simulink model "PC_MSFS_STATION"  (R2021b)
settings: Solver=FixedStepAuto  StartTime=0.0  StopTime=700  FixedStep=0.03  RelTol=1e-3
undefined symbols (not defined in the file): DiscIntNeverNeededParam, f, MODEL, MODEL_INI
libraries: SimConnectToolbox x13, simulink x5, instrumentlib x3
(part 1 of 2)
settings Model: Creator=Andreas  LastModifiedBy=ae-dagbeyibor3
settings SolverCC: AlgebraicLoopSolver=TrustRegion
settings DebuggingCC: InheritedTsInSrcMsg=none  SFMachineParentedDataDiag=warning

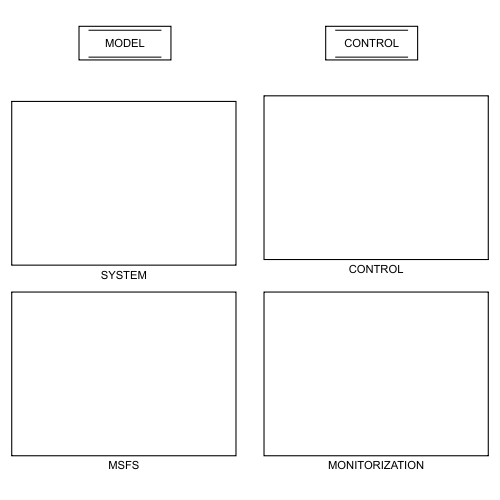
[thumbnail: Simulink's stored preview of the top-level diagram]
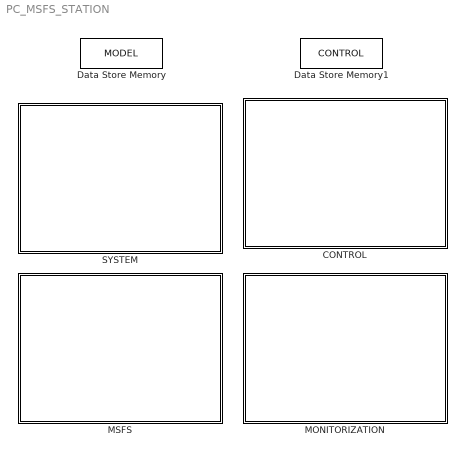
== system PC_MSFS_STATION ==
  CONTROL : Subsystem
  Data Store Memory : DataStoreMemory  DataStoreName=MODEL  ReadBeforeWriteMsg=warning  WriteAfterWriteMsg=warning  WriteAfterReadMsg=warning  InitialValue=MODEL_INI  ShowAdditionalParam=off  OutDataTypeStr=Bus: MODEL_Bus
  Data Store Memory1 : DataStoreMemory  DataStoreName=CONTROL  ReadBeforeWriteMsg=warning  WriteAfterWriteMsg=warning  WriteAfterReadMsg=warning  InitialValue=CONTROL_INI  ShowAdditionalParam=off  OutDataTypeStr=Bus: CONTROL_Bus
  MONITORIZATION : Subsystem
  MSFS : Subsystem
  SYSTEM : Subsystem

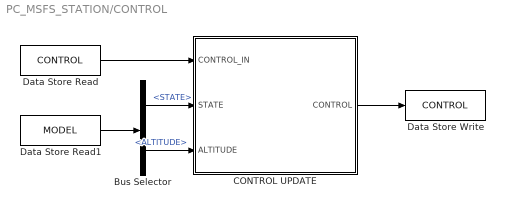
== system PC_MSFS_STATION/CONTROL ==
  Bus Selector : BusSelector  OutputSignals=STATE,INPUT.ALTITUDE
  CONTROL UPDATE : MATLAB Function  TreatAsAtomicUnit=on
  Data Store Read : DataStoreRead  DataStoreName=CONTROL  SampleTime=MODEL_INI.PARAM.SIM_SAMPLING_TIME  IndexOptions=Index vector (dialog)  Indices=1  OutputSizes=1
  Data Store Read1 : DataStoreRead  DataStoreName=MODEL  SampleTime=MODEL_INI.PARAM.SIM_SAMPLING_TIME  IndexOptions=Index vector (dialog)  Indices=1  OutputSizes=1
  Data Store Write : DataStoreWrite  DataStoreName=CONTROL  IndexOptions=Index vector (dialog)  Indices=1  OutputSizes=1
  wires:
  Data Store Read/1 -> CONTROL UPDATE/1(CONTROL_IN)
  CONTROL UPDATE/1(CONTROL) -> Data Store Write/1
  Bus Selector/1 -> CONTROL UPDATE/2(STATE)  "<STATE>"
  Data Store Read1/1 -> Bus Selector/1
  Bus Selector/2 -> CONTROL UPDATE/3(ALTITUDE)  "<ALTITUDE>"

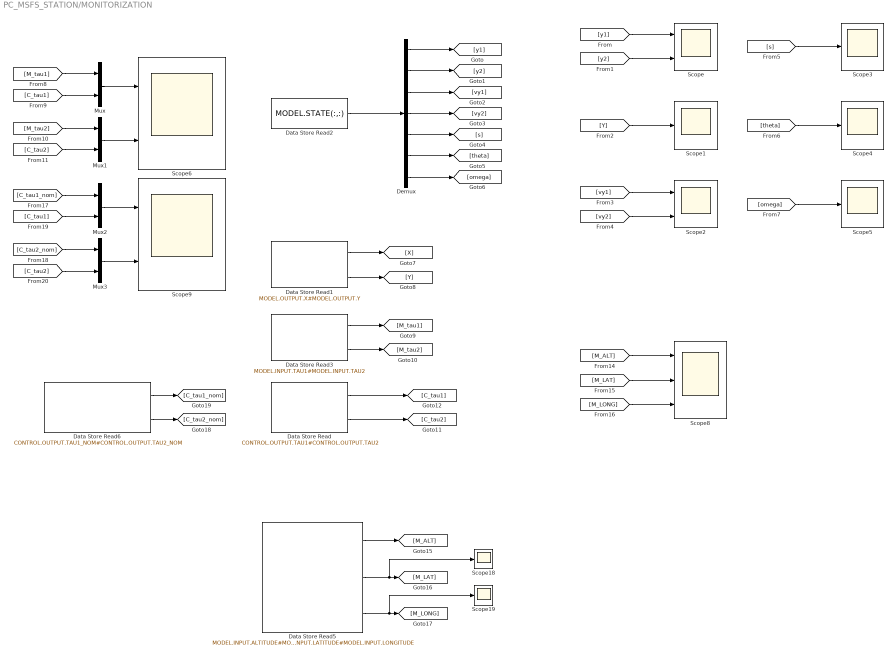
== system PC_MSFS_STATION/MONITORIZATION ==
  Data Store Read : DataStoreRead  DataStoreName=CONTROL  DataStoreElements=CONTROL.OUTPUT.TAU1#CONTROL.OUTPUT.TAU2  IndexOptions=Index vector (dialog)  Indices=1  OutputSizes=1
  Data Store Read1 : DataStoreRead  DataStoreName=MODEL  SampleTime=MODEL_INI.PARAM.SIM_SAMPLING_TIME  DataStoreElements=MODEL.OUTPUT.X#MODEL.OUTPUT.Y  IndexOptions=Index vector (dialog)  Indices=1  OutputSizes=1
  Data Store Read2 : DataStoreRead  DataStoreName=MODEL  SampleTime=MODEL_INI.PARAM.SIM_SAMPLING_TIME  DataStoreElements=MODEL.STATE(:,:)  IndexOptions=Index vector (dialog)  Indices=1  OutputSizes=1
  Data Store Read3 : DataStoreRead  DataStoreName=MODEL  SampleTime=MODEL_INI.PARAM.SIM_SAMPLING_TIME  DataStoreElements=MODEL.INPUT.TAU1#MODEL.INPUT.TAU2  IndexOptions=Index vector (dialog)  Indices=1  OutputSizes=1
  Data Store Read5 : DataStoreRead  DataStoreName=MODEL  SampleTime=MODEL_INI.PARAM.SIM_SAMPLING_TIME  DataStoreElements=MODEL.INPUT.ALTITUDE#MODEL.INPUT.LATITUDE#MODEL.INPUT.LONGITUDE  IndexOptions=Index vector (dialog)  Indices=1  OutputSizes=1
  Data Store Read6 : DataStoreRead  DataStoreName=CONTROL  DataStoreElements=CONTROL.OUTPUT.TAU1_NOM#CONTROL.OUTPUT.TAU2_NOM  IndexOptions=Index vector (dialog)  Indices=1  OutputSizes=1
  Demux : Demux  Outputs=7
  Mux{,1..3} (4 alike) : Mux  Inputs=2
  Scope{,2,6,9} (4 alike) : Scope  NumInputPorts=2
  Scope{1,3..5,18..19} (6 alike) : Scope
  Scope8 : Scope  NumInputPorts=3
  wires:
  Data Store Read2/1 -> Demux/1
  Demux/1 -> [y1]
  Demux/2 -> [y2]
  Demux/3 -> [vy1]
  Demux/4 -> [vy2]
  Demux/5 -> [s]
  Demux/6 -> [theta]
  Demux/7 -> [omega]
  [y1] -> Scope/1
  [y2] -> Scope/2
  Data Store Read1/1 -> [X]
  Data Store Read1/2 -> [Y]
  [Y] -> Scope1/1
  [vy2] -> Scope2/2
  [vy1] -> Scope2/1
  [s] -> Scope3/1
  [theta] -> Scope4/1
  [omega] -> Scope5/1
  Data Store Read3/1 -> [M_tau1]
  Data Store Read3/2 -> [M_tau2]
  Data Store Read/1 -> [C_tau1]
  Data Store Read/2 -> [C_tau2]
  Mux/1 -> Scope6/1
  Mux1/1 -> Scope6/2
  [M_tau1] -> Mux/1
  [M_tau2] -> Mux1/1
  [C_tau2] -> Mux1/2
  [C_tau1] -> Mux/2
  Data Store Read5/2 -> Scope18/1, [M_LAT]
  Data Store Read5/1 -> [M_ALT]
  Data Store Read5/3 -> Scope19/1, [M_LONG]
  [M_LAT] -> Scope8/2
  [M_ALT] -> Scope8/1
  [M_LONG] -> Scope8/3
  Data Store Read6/2 -> [C_tau2_nom]
  Data Store Read6/1 -> [C_tau1_nom]
  [C_tau1] -> Mux2/2
  [C_tau2] -> Mux3/2
  [C_tau2_nom] -> Mux3/1
  [C_tau1_nom] -> Mux2/1
  Mux3/1 -> Scope9/2
  Mux2/1 -> Scope9/1

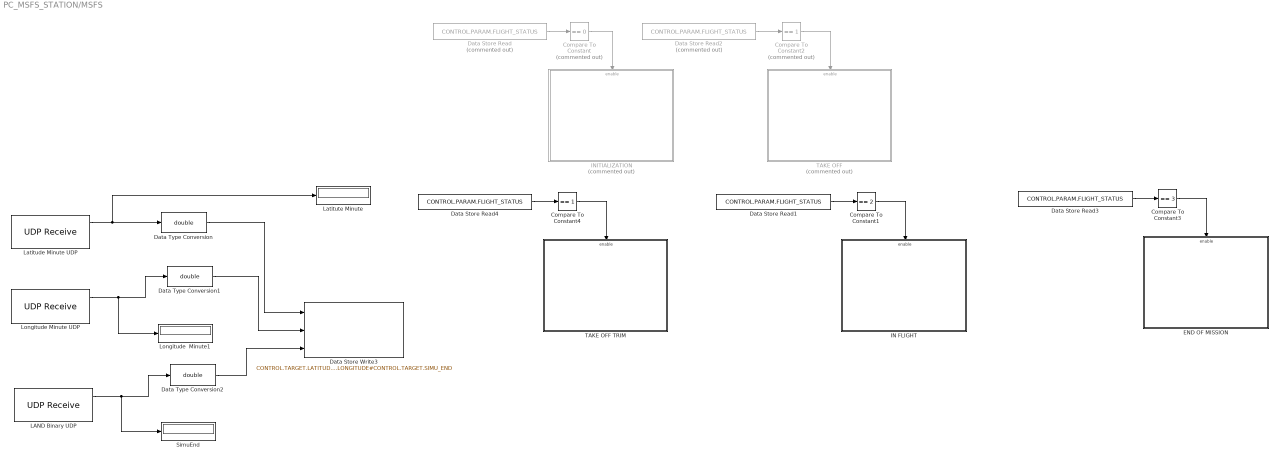
== system PC_MSFS_STATION/MSFS ==
  Compare To Constant : simulink/Logic and Bit Operations/Compare To Constant  Commented=on  relop===  const=0  OutDataTypeStr=boolean
  Compare To Constant1 : simulink/Logic and Bit Operations/Compare To Constant  relop===  const=2  OutDataTypeStr=boolean
  Compare To Constant2 : simulink/Logic and Bit Operations/Compare To Constant  Commented=on  relop===  const=1  OutDataTypeStr=boolean
  Compare To Constant3 : simulink/Logic and Bit Operations/Compare To Constant  relop===  const=3  OutDataTypeStr=boolean
  Compare To Constant4 : simulink/Logic and Bit Operations/Compare To Constant  relop===  const=1  OutDataTypeStr=boolean
  Data Store Read : DataStoreRead  Commented=on  DataStoreName=CONTROL  DataStoreElements=CONTROL.PARAM.FLIGHT_STATUS  IndexOptions=Index vector (dialog)  Indices=1  OutputSizes=1
  Data Store Read1 : DataStoreRead  DataStoreName=CONTROL  DataStoreElements=CONTROL.PARAM.FLIGHT_STATUS  IndexOptions=Index vector (dialog)  Indices=1  OutputSizes=1
  Data Store Read2 : DataStoreRead  Commented=on  DataStoreName=CONTROL  DataStoreElements=CONTROL.PARAM.FLIGHT_STATUS  IndexOptions=Index vector (dialog)  Indices=1  OutputSizes=1
  Data Store Read3 : DataStoreRead  DataStoreName=CONTROL  DataStoreElements=CONTROL.PARAM.FLIGHT_STATUS  IndexOptions=Index vector (dialog)  Indices=1  OutputSizes=1
  Data Store Read4 : DataStoreRead  DataStoreName=CONTROL  DataStoreElements=CONTROL.PARAM.FLIGHT_STATUS  IndexOptions=Index vector (dialog)  Indices=1  OutputSizes=1
  Data Store Write3 : DataStoreWrite  DataStoreName=CONTROL  DataStoreElements=CONTROL.TARGET.LATITUDE#CONTROL.TARGET.LONGITUDE#CONTROL.TARGET.SIMU_END  IndexOptions=Index vector (dialog)  Indices=1  OutputSizes=1
  Data Type Conversion : DataTypeConversion  OutDataTypeStr=double
  Data Type Conversion1 : DataTypeConversion  OutDataTypeStr=double
  Data Type Conversion2 : DataTypeConversion  OutDataTypeStr=double
  END OF MISSION : Subsystem
  IN FLIGHT : Subsystem
  INITIALIZATION : Subsystem  Commented=on
  LAND Binary UDP : instrumentlib/UDP Receive  Priority=1  Host=127.0.0.1  Port=8081  LocalPort=8086  EnablePortSharing=off  GetLatestData=off  DataSize=[1 1]  DataType=single  ASCIIFormatting=%f,  Terminator=LF  ByteOrder=BigEndian  EnableBlockingMode=off  Timeout=5  SampleTime=0.03  LocalAddress=127.0.0.1
  Latitude Minute UDP : instrumentlib/UDP Receive  Priority=1  Host=127.0.0.1  Port=8081  LocalPort=8082  EnablePortSharing=off  GetLatestData=off  DataSize=[1 1]  DataType=single  ASCIIFormatting=%f,  Terminator=LF  ByteOrder=BigEndian  EnableBlockingMode=off  Timeout=5  SampleTime=0.03  LocalAddress=127.0.0.1
  Latitute Minute : Display
  Longitude  Minute1 : Display
  Longitude Minute UDP : instrumentlib/UDP Receive  Priority=1  Host=127.0.0.1  Port=8081  LocalPort=8084  EnablePortSharing=off  GetLatestData=off  DataSize=[1 1]  DataType=single  ASCIIFormatting=%f,  Terminator=LF  ByteOrder=BigEndian  EnableBlockingMode=off  Timeout=5  SampleTime=0.03  LocalAddress=127.0.0.1
  SimuEnd : Display
  TAKE OFF : Subsystem  Commented=on
  TAKE OFF TRIM : Subsystem
  wires:
  Data Store Read/1 -> Compare To Constant/1
  Compare To Constant/1 -> INITIALIZATION/Enable
  Data Store Read1/1 -> Compare To Constant1/1
  Compare To Constant1/1 -> IN FLIGHT/Enable
  Data Store Read2/1 -> Compare To Constant2/1
  Compare To Constant2/1 -> TAKE OFF/Enable
  Compare To Constant3/1 -> END OF MISSION/Enable
  Data Store Read3/1 -> Compare To Constant3/1
  Data Store Read4/1 -> Compare To Constant4/1
  Compare To Constant4/1 -> TAKE OFF TRIM/Enable
  Longitude Minute UDP/1 -> Longitude  Minute1/1, Data Type Conversion1/1
  Data Type Conversion/1 -> Data Store Write3/1
  Latitude Minute UDP/1 -> Latitute Minute/1, Data Type Conversion/1
  Data Type Conversion1/1 -> Data Store Write3/2
  LAND Binary UDP/1 -> SimuEnd/1, Data Type Conversion2/1
  Data Type Conversion2/1 -> Data Store Write3/3

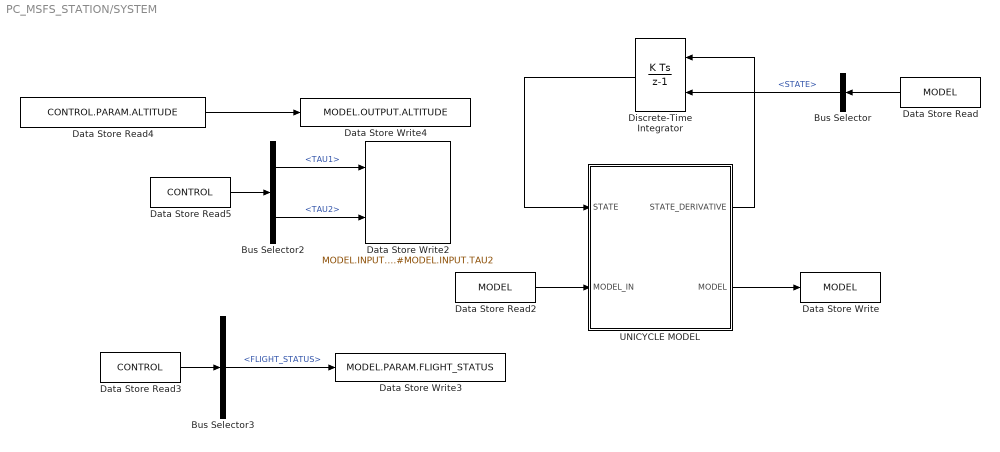
== system PC_MSFS_STATION/SYSTEM ==
  Bus Selector : BusSelector  OutputSignals=STATE
  Bus Selector2 : BusSelector  OutputSignals=OUTPUT.TAU1,OUTPUT.TAU2
  Bus Selector3 : BusSelector  OutputSignals=PARAM.FLIGHT_STATUS
  Data Store Read : DataStoreRead  DataStoreName=MODEL  SampleTime=MODEL_INI.PARAM.SIM_SAMPLING_TIME  IndexOptions=Index vector (dialog)  Indices=1  OutputSizes=1
  Data Store Read2 : DataStoreRead  DataStoreName=MODEL  SampleTime=MODEL_INI.PARAM.SIM_SAMPLING_TIME  IndexOptions=Index vector (dialog)  Indices=1  OutputSizes=1
  Data Store Read3 : DataStoreRead  DataStoreName=CONTROL  IndexOptions=Index vector (dialog)  Indices=1  OutputSizes=1
  Data Store Read4 : DataStoreRead  DataStoreName=CONTROL  DataStoreElements=CONTROL.PARAM.ALTITUDE  IndexOptions=Index vector (dialog)  Indices=1  OutputSizes=1
  Data Store Read5 : DataStoreRead  DataStoreName=CONTROL  IndexOptions=Index vector (dialog)  Indices=1  OutputSizes=1
  Data Store Write : DataStoreWrite  DataStoreName=MODEL  IndexOptions=Index vector (dialog)  Indices=1  OutputSizes=1
  Data Store Write2 : DataStoreWrite  DataStoreName=MODEL  DataStoreElements=MODEL.INPUT.TAU1#MODEL.INPUT.TAU2  IndexOptions=Index vector (dialog)  Indices=1  OutputSizes=1
  Data Store Write3 : DataStoreWrite  DataStoreName=MODEL  DataStoreElements=MODEL.PARAM.FLIGHT_STATUS  IndexOptions=Index vector (dialog)  Indices=1  OutputSizes=1
  Data Store Write4 : DataStoreWrite  DataStoreName=MODEL  DataStoreElements=MODEL.OUTPUT.ALTITUDE  IndexOptions=Index vector (dialog)  Indices=1  OutputSizes=1
  Discrete-Time Integrator : DiscreteIntegrator  InitialConditionSource=external  SampleTime=-1  ICPrevOutput=DiscIntNeverNeededParam  ICPrevScaledInput=DiscIntNeverNeededParam
  UNICYCLE MODEL : MATLAB Function  TreatAsAtomicUnit=on
  wires:
  Discrete-Time Integrator/1 -> UNICYCLE MODEL/1(STATE)
  UNICYCLE MODEL/1(STATE_DERIVATIVE) -> Discrete-Time Integrator/1
  Bus Selector/1 -> Discrete-Time Integrator/2  "<STATE>"
  Data Store Read/1 -> Bus Selector/1
  Data Store Read2/1 -> UNICYCLE MODEL/2(MODEL_IN)
  UNICYCLE MODEL/2(MODEL) -> Data Store Write/1
  Bus Selector2/2 -> Data Store Write2/2  "<TAU2>"
  Bus Selector2/1 -> Data Store Write2/1  "<TAU1>"
  Data Store Read5/1 -> Bus Selector2/1
  Data Store Read3/1 -> Bus Selector3/1
  Bus Selector3/1 -> Data Store Write3/1  "<FLIGHT_STATUS>"
  Data Store Read4/1 -> Data Store Write4/1

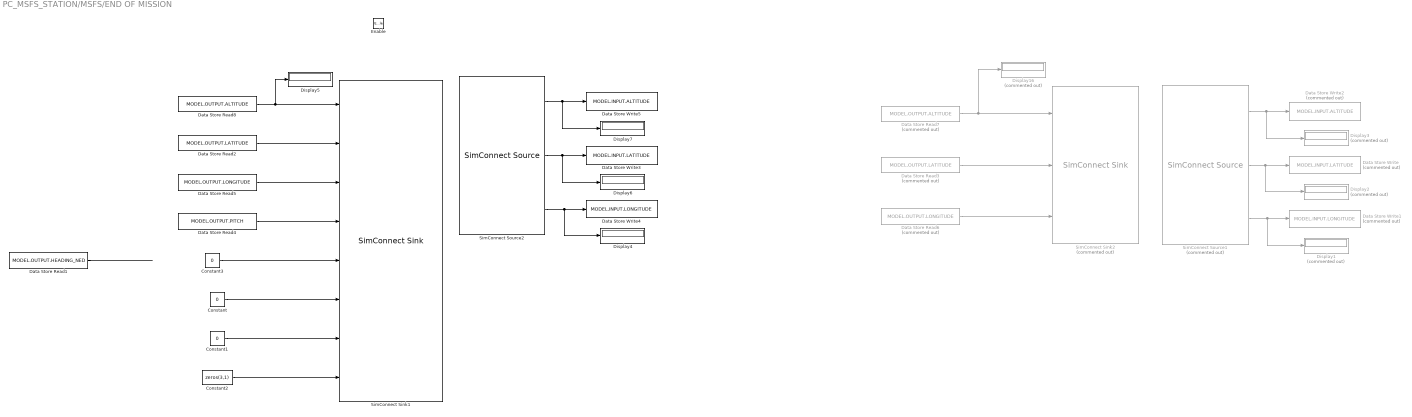
== system PC_MSFS_STATION/MSFS/END OF MISSION ==
  Enable : EnablePort
  Constant : Constant  Value=0  SampleTime=-1
  Constant1 : Constant  Value=0  SampleTime=-1
  Constant2 : Constant  Value=zeros(3,1)  SampleTime=-1
  Constant3 : Constant  Value=0  SampleTime=-1
  Data Store Read1 : DataStoreRead  DataStoreName=MODEL  DataStoreElements=MODEL.OUTPUT.HEADING_NED  IndexOptions=Index vector (dialog)  Indices=1  OutputSizes=1
  Data Store Read2 : DataStoreRead  DataStoreName=MODEL  DataStoreElements=MODEL.OUTPUT.LATITUDE  IndexOptions=Index vector (dialog)  Indices=1  OutputSizes=1
  Data Store Read3 : DataStoreRead  Commented=on  DataStoreName=MODEL  DataStoreElements=MODEL.OUTPUT.LATITUDE  IndexOptions=Index vector (dialog)  Indices=1  OutputSizes=1
  Data Store Read4 : DataStoreRead  DataStoreName=MODEL  DataStoreElements=MODEL.OUTPUT.PITCH  IndexOptions=Index vector (dialog)  Indices=1  OutputSizes=1
  Data Store Read5 : DataStoreRead  DataStoreName=MODEL  DataStoreElements=MODEL.OUTPUT.LONGITUDE  IndexOptions=Index vector (dialog)  Indices=1  OutputSizes=1
  Data Store Read6 : DataStoreRead  Commented=on  DataStoreName=MODEL  DataStoreElements=MODEL.OUTPUT.LONGITUDE  IndexOptions=Index vector (dialog)  Indices=1  OutputSizes=1
  Data Store Read7 : DataStoreRead  Commented=on  DataStoreName=MODEL  DataStoreElements=MODEL.OUTPUT.ALTITUDE  IndexOptions=Index vector (dialog)  Indices=1  OutputSizes=1
  Data Store Read8 : DataStoreRead  DataStoreName=MODEL  DataStoreElements=MODEL.OUTPUT.ALTITUDE  IndexOptions=Index vector (dialog)  Indices=1  OutputSizes=1
  Data Store Write : DataStoreWrite  Commented=on  DataStoreName=MODEL  DataStoreElements=MODEL.INPUT.LATITUDE  IndexOptions=Index vector (dialog)  Indices=1  OutputSizes=1
  Data Store Write1 : DataStoreWrite  Commented=on  DataStoreName=MODEL  DataStoreElements=MODEL.INPUT.LONGITUDE  IndexOptions=Index vector (dialog)  Indices=1  OutputSizes=1
  Data Store Write2 : DataStoreWrite  Commented=on  DataStoreName=MODEL  DataStoreElements=MODEL.INPUT.ALTITUDE  IndexOptions=Index vector (dialog)  Indices=1  OutputSizes=1
  Data Store Write3 : DataStoreWrite  DataStoreName=MODEL  DataStoreElements=MODEL.INPUT.LATITUDE  IndexOptions=Index vector (dialog)  Indices=1  OutputSizes=1
  Data Store Write4 : DataStoreWrite  DataStoreName=MODEL  DataStoreElements=MODEL.INPUT.LONGITUDE  IndexOptions=Index vector (dialog)  Indices=1  OutputSizes=1
  Data Store Write5 : DataStoreWrite  DataStoreName=MODEL  DataStoreElements=MODEL.INPUT.ALTITUDE  IndexOptions=Index vector (dialog)  Indices=1  OutputSizes=1
  Display{1..3,16} (4 alike) : Display  Commented=on
  Display{4..7} (4 alike) : Display
  SimConnect Sink1 : SimConnectToolbox/SimConnect Sink  configurationIndex=0  connectionName=SimConnectSink  variables=|
      | PLANE ALTITUDE, FEET;
      | PLANE LATITUDE, RADIANS;
      | PLANE LONGITUDE, RADIANS;
      | PLANE PITCH DEGREES, RADIANS;
      | PLANE HEADING DEGREES TRUE, RADIANS;
      | ROTATION VELOCITY BODY X, FEET PER SECOND;
      | AILERON POSITION, POSITION;
      | AILERON TRIM PCT, PERCENT;
      settings: SourceProductName=SimConnect Toolbox
      mask Display:
      | % This is a new mask on top of the base mask.
      | % Use "View base mask" link below to see the base mask.
      | %port_label('input', 1, 'Rudder Trim', 'texmode', 'on')
      | port_label('input', 1, 'PLANE ALTITUDE, FEET', 'texmode', 'on')
      | port_label('input', 2, 'PLANE LATITUDE, RADIANS', 'texmode', 'on')
      | port_label('input', 3, 'PLANE LONGITUDE, RADIANS', 'texmode', 'on')
      | port_label('input', 4, 'PITCH DEGREES, RADIANS', 'texmode', 'on')
      | port_label('input', 5, 'HEADING DEGREES TRUE, RADIANS', 'texmode', 'on')
      | port_label('input', 6, 'VELOCITY BODY X, FEET PER SECOND', 'texmode', 'on')
      | port_label('input', 7, 'AILERON POSITION, POSITION', 'texmode', 'on')
      | port_label('input', 8, 'AILERON TRIM PCT, PERCENT OVER 100', 'texmode', 'on')
  SimConnect Sink2 : SimConnectToolbox/SimConnect Sink  Commented=on  configurationIndex=0  connectionName=SimConnectSink  variables=|
      | PLANE ALTITUDE, FEET;
      | PLANE LATITUDE, RADIANS;
      | PLANE LONGITUDE, RADIANS;
      settings: SourceProductName=SimConnect Toolbox
      mask Display:
      | % This is a new mask on top of the base mask.
      | % Use "View base mask" link below to see the base mask.
      | %port_label('input', 1, 'Rudder Trim', 'texmode', 'on')
      | port_label('input', 1, 'PLANE ALTITUDE, FEET', 'texmode', 'on')
      | port_label('input', 2, 'PLANE LATITUDE, RADIANS', 'texmode', 'on')
      | port_label('input', 3, 'PLANE LONGITUDE, RADIANS', 'texmode', 'on')
  SimConnect Source1 : SimConnectToolbox/SimConnect Source  Commented=on  configurationIndex=0  connectionName=SimConnectSource  variables=|
      | PLANE ALTITUDE, FEET;
      | PLANE LATITUDE, RADIANS;
      | PLANE LONGITUDE, RADIANS;
      settings: SourceProductName=SimConnect Toolbox
      mask Display:
      | % This is a new mask on top of the base mask.
      | % Use "View base mask" link below to see the base mask.
      | % port_label('output', 1, 'g', 'texmode', 'on')
      | port_label('output', 1, 'PLANE ALTITUDE, FEET', 'texmode', 'on')
      | port_label('output', 2, 'PLANE LATITUDE, RADIANS', 'texmode', 'on')
      | port_label('output', 3, 'PLANE LONGITUDE, RADIANS', 'texmode', 'on')
  SimConnect Source2 : SimConnectToolbox/SimConnect Source  configurationIndex=0  connectionName=SimConnectSource  variables=|
      | PLANE ALTITUDE, FEET;
      | PLANE LATITUDE, RADIANS;
      | PLANE LONGITUDE, RADIANS;
      settings: SourceProductName=SimConnect Toolbox
      mask Display:
      | % This is a new mask on top of the base mask.
      | % Use "View base mask" link below to see the base mask.
      | % port_label('output', 1, 'g', 'texmode', 'on')
      | port_label('output', 1, 'PLANE ALTITUDE, FEET', 'texmode', 'on')
      | port_label('output', 2, 'PLANE LATITUDE, RADIANS', 'texmode', 'on')
      | port_label('output', 3, 'PLANE LONGITUDE, RADIANS', 'texmode', 'on')
  wires:
  SimConnect Source1/3 -> Data Store Write1/1, Display1/1
  SimConnect Source1/1 -> Data Store Write2/1, Display3/1
  SimConnect Source1/2 -> Display2/1, Data Store Write/1
  Data Store Read7/1 -> Display16/1, SimConnect Sink2/1
  Data Store Read6/1 -> SimConnect Sink2/3
  Data Store Read3/1 -> SimConnect Sink2/2
  SimConnect Source2/1 -> Display7/1, Data Store Write5/1
  Data Store Read5/1 -> SimConnect Sink1/3
  Data Store Read2/1 -> SimConnect Sink1/2
  Data Store Read8/1 -> SimConnect Sink1/1, Display5/1
  SimConnect Source2/2 -> Data Store Write3/1, Display6/1
  Data Store Read4/1 -> SimConnect Sink1/4
  SimConnect Source2/3 -> Display4/1, Data Store Write4/1
  Constant1/1 -> SimConnect Sink1/7
  Data Store Read1/1 -> ?
  Constant2/1 -> SimConnect Sink1/8
  Constant/1 -> SimConnect Sink1/6
  Constant3/1 -> SimConnect Sink1/5

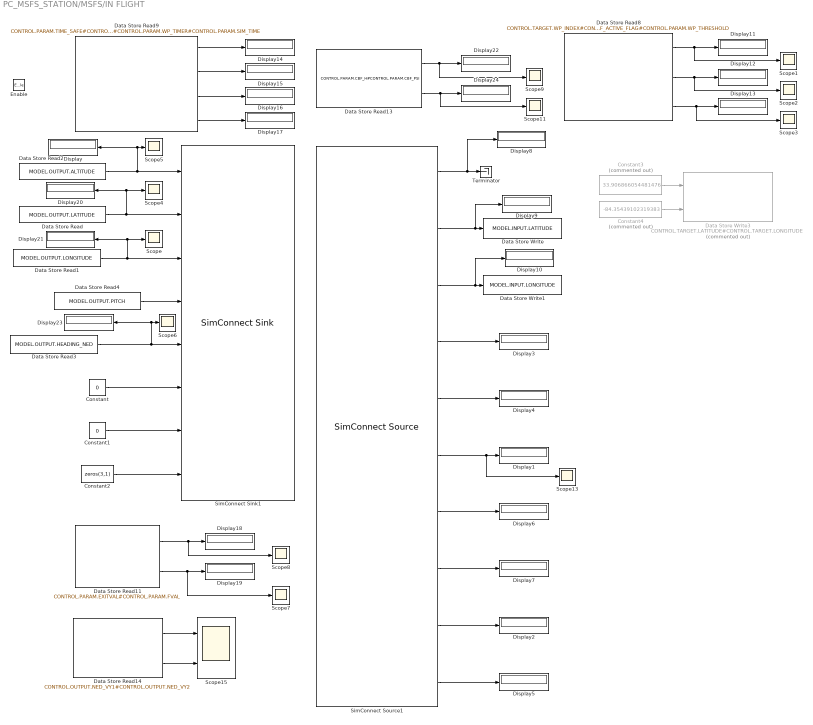
== system PC_MSFS_STATION/MSFS/IN FLIGHT ==
  Enable : EnablePort
  Constant : Constant  Value=0  SampleTime=-1
  Constant1 : Constant  Value=0  SampleTime=-1
  Constant2 : Constant  Value=zeros(3,1)  SampleTime=-1
  Constant3 : Constant  Commented=on  Value=33.906866054481476  SampleTime=-1
  Constant4 : Constant  Commented=on  Value=-84.35439102319383  SampleTime=-1
  Data Store Read : DataStoreRead  DataStoreName=MODEL  DataStoreElements=MODEL.OUTPUT.LATITUDE  IndexOptions=Index vector (dialog)  Indices=1  OutputSizes=1
  Data Store Read1 : DataStoreRead  DataStoreName=MODEL  DataStoreElements=MODEL.OUTPUT.LONGITUDE  IndexOptions=Index vector (dialog)  Indices=1  OutputSizes=1
  Data Store Read11 : DataStoreRead  DataStoreName=CONTROL  DataStoreElements=CONTROL.PARAM.EXITVAL#CONTROL.PARAM.FVAL  IndexOptions=Index vector (dialog)  Indices=1  OutputSizes=1
  Data Store Read13 : DataStoreRead  DataStoreName=CONTROL  DataStoreElements=CONTROL.PARAM.CBF_H#CONTROL.PARAM.CBF_PSI  IndexOptions=Index vector (dialog)  Indices=1  OutputSizes=1
  Data Store Read14 : DataStoreRead  DataStoreName=CONTROL  DataStoreElements=CONTROL.OUTPUT.NED_VY1#CONTROL.OUTPUT.NED_VY2  IndexOptions=Index vector (dialog)  Indices=1  OutputSizes=1
  Data Store Read2 : DataStoreRead  DataStoreName=MODEL  DataStoreElements=MODEL.OUTPUT.ALTITUDE  IndexOptions=Index vector (dialog)  Indices=1  OutputSizes=1
  Data Store Read3 : DataStoreRead  DataStoreName=MODEL  DataStoreElements=MODEL.OUTPUT.HEADING_NED  IndexOptions=Index vector (dialog)  Indices=1  OutputSizes=1
  Data Store Read4 : DataStoreRead  DataStoreName=MODEL  DataStoreElements=MODEL.OUTPUT.PITCH  IndexOptions=Index vector (dialog)  Indices=1  OutputSizes=1
  Data Store Read8 : DataStoreRead  DataStoreName=CONTROL  DataStoreElements=CONTROL.TARGET.WP_INDEX#CONTROL.PARAM.CBF_ACTIVE_FLAG#CONTROL.PARAM.WP_THRESHOLD  IndexOptions=Index vector (dialog)  Indices=1  OutputSizes=1
  Data Store Read9 : DataStoreRead  DataStoreName=CONTROL  DataStoreElements=CONTROL.PARAM.TIME_SAFE#CONTROL.PARAM.TIMER#CONTROL.PARAM.WP_TIMER#CONTROL.PARAM.SIM_TIME  IndexOptions=Index vector (dialog)  Indices=1  OutputSizes=1
  Data Store Write : DataStoreWrite  DataStoreName=MODEL  DataStoreElements=MODEL.INPUT.LATITUDE  IndexOptions=Index vector (dialog)  Indices=1  OutputSizes=1
  Data Store Write1 : DataStoreWrite  DataStoreName=MODEL  DataStoreElements=MODEL.INPUT.LONGITUDE  IndexOptions=Index vector (dialog)  Indices=1  OutputSizes=1
  Data Store Write3 : DataStoreWrite  Commented=on  DataStoreName=CONTROL  DataStoreElements=CONTROL.TARGET.LATITUDE#CONTROL.TARGET.LONGITUDE  IndexOptions=Index vector (dialog)  Indices=1  OutputSizes=1
  Display{,1..24} (25 alike) : Display
  Scope{,1..9,11,13} (12 alike) : Scope
  Scope15 : Scope  NumInputPorts=2
  SimConnect Sink1 : SimConnectToolbox/SimConnect Sink  configurationIndex=0  connectionName=SimConnectSink  variables=|
      | PLANE ALTITUDE, FEET;
      | PLANE LATITUDE, RADIANS;
      | PLANE LONGITUDE, RADIANS;
      | PLANE PITCH DEGREES, RADIANS;
      | PLANE HEADING DEGREES TRUE, RADIANS;
      | ROTATION VELOCITY BODY X, FEET PER SECOND;
      | AILERON POSITION, POSITION;
      | AILERON TRIM PCT, PERCENT;
      settings: SourceProductName=SimConnect Toolbox
      mask Display:
      | % This is a new mask on top of the base mask.
      | % Use "View base mask" link below to see the base mask.
      | %port_label('input', 1, 'Rudder Trim', 'texmode', 'on')
      | port_label('input', 1, 'PLANE ALTITUDE, FEET', 'texmode', 'on')
      | port_label('input', 2, 'PLANE LATITUDE, RADIANS', 'texmode', 'on')
      | port_label('input', 3, 'PLANE LONGITUDE, RADIANS', 'texmode', 'on')
      | port_label('input', 4, 'PITCH DEGREES, RADIANS', 'texmode', 'on')
      | port_label('input', 5, 'HEADING DEGREES TRUE, RADIANS', 'texmode', 'on')
      | port_label('input', 6, 'VELOCITY BODY X, FEET PER SECOND', 'texmode', 'on')
      | port_label('input', 7, 'AILERON POSITION, POSITION', 'texmode', 'on')
      | port_label('input', 8, 'AILERON TRIM PCT, PERCENT OVER 100', 'texmode', 'on')
  SimConnect Source1 : SimConnectToolbox/SimConnect Source  configurationIndex=0  connectionName=SimConnectSource  variables=|
      | PLANE ALTITUDE, FEET;
      | PLANE LATITUDE, RADIANS;
      | PLANE LONGITUDE, RADIANS;
      | ROTATION VELOCITY BODY X, FEET PER SECOND;
      | PLANE PITCH DEGREES, RADIANS;
      | PLANE HEADING DEGREES TRUE, RADIANS;
      | PLANE HEADING DEGREES MAGNETIC, RADIANS;
      | PLANE HEADING DEGREES GYRO, DEGREES;
      | AILERON POSITION, POSITION;
      | AILERON TRIM PCT, PERCENT OVER 100;
      settings: SourceProductName=SimConnect Toolbox
      mask Display:
      | % This is a new mask on top of the base mask.
      | % Use "View base mask" link below to see the base mask.
      | % port_label('output', 1, 'g', 'texmode', 'on')
      | port_label('output', 1, 'PLANE ALTITUDE, FEET', 'texmode', 'on')
      | port_label('output', 2, 'PLANE LATITUDE, RADIANS', 'texmode', 'on')
      | port_label('output', 3, 'PLANE LONGITUDE, RADIANS', 'texmode', 'on')
      | port_label('output', 4, 'VELOCITY BODY X, FEET PER SECOND', 'texmode', 'on')
      | port_label('output', 5, 'PITCH DEGREES, RADIANS', 'texmode', 'on')
      | port_label('output', 6, 'HEADING DEGREES TRUE, RADIANS', 'texmode', 'on')
      | port_label('output', 7, 'HEADING DEGREES MAGNETIC, RADIANS', 'texmode', 'on')
      | port_label('output', 8, 'HEADING DEGREES GYRO, DEGREES', 'texmode', 'on')
      | port_label('output', 9, 'AILERON POSITION, POSITION', 'texmode', 'on')
      | port_label('output', 10, 'AILERON TRIM PCT, PERCENT OVER 100', 'texmode', 'on')
  Terminator : Terminator
  wires:
  Constant2/1 -> SimConnect Sink1/8
  SimConnect Source1/9 -> Display2/1
  Constant/1 -> SimConnect Sink1/6
  Data Store Read1/1 -> Display21/1, Scope/1, SimConnect Sink1/3
  Constant1/1 -> SimConnect Sink1/7
  SimConnect Source1/5 -> Display4/1
  SimConnect Source1/3 -> Display10/1, Data Store Write1/1
  SimConnect Source1/2 -> Display9/1, Data Store Write/1
  SimConnect Source1/8 -> Display7/1
  SimConnect Source1/6 -> Scope13/1, Display1/1
  Data Store Read2/1 -> Display/1, Scope5/1, SimConnect Sink1/1
  Data Store Read/1 -> Display20/1, Scope4/1, SimConnect Sink1/2
  Data Store Read4/1 -> SimConnect Sink1/4
  SimConnect Source1/4 -> Display3/1
  SimConnect Source1/1 -> Terminator/1, Display8/1
  SimConnect Source1/7 -> Display6/1
  SimConnect Source1/10 -> Display5/1
  Data Store Read9/1 -> Display14/1
  Data Store Read9/2 -> Display15/1
  Data Store Read9/3 -> Display16/1
  Data Store Read9/4 -> Display17/1
  Data Store Read13/1 -> Scope9/1, Display22/1
  Data Store Read13/2 -> Scope11/1, Display24/1
  Data Store Read14/1 -> Scope15/1
  Data Store Read14/2 -> Scope15/2
  Data Store Read11/1 -> Scope8/1, Display18/1
  Data Store Read11/2 -> Scope7/1, Display19/1
  Data Store Read8/1 -> Scope1/1, Display11/1
  Data Store Read8/2 -> Display12/1, Scope2/1
  Data Store Read8/3 -> Display13/1, Scope3/1
  Constant3/1 -> Data Store Write3/1
  Constant4/1 -> Data Store Write3/2
  Data Store Read3/1 -> Display23/1, Scope6/1, SimConnect Sink1/5

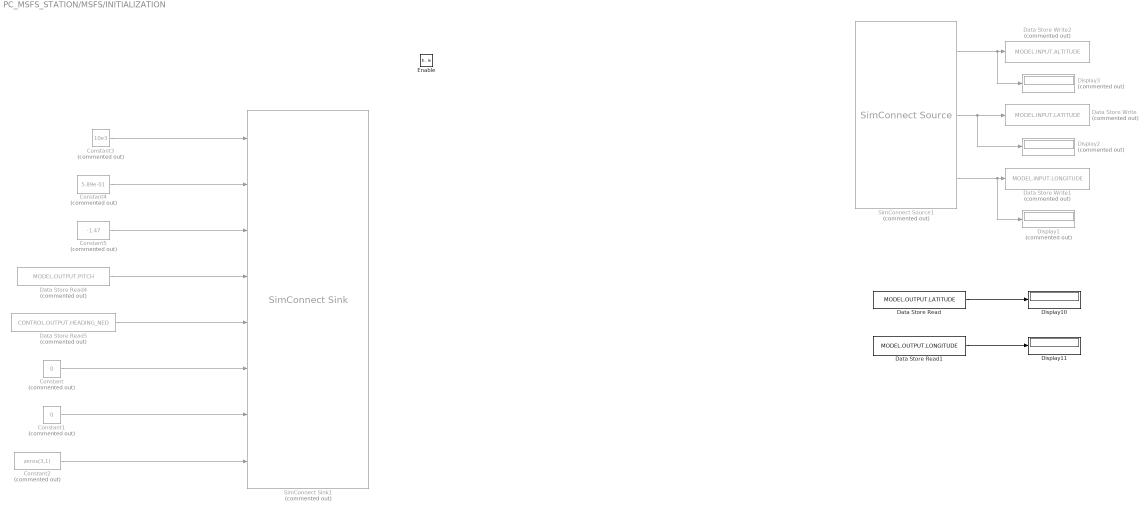
== system PC_MSFS_STATION/MSFS/INITIALIZATION ==
  Enable : EnablePort
  Constant : Constant  Commented=on  Value=0  SampleTime=-1
  Constant1 : Constant  Commented=on  Value=0  SampleTime=-1
  Constant2 : Constant  Commented=on  Value=zeros(3,1)  SampleTime=-1
  Constant3 : Constant  Commented=on  Value=10e3  SampleTime=-1
  Constant4 : Constant  Commented=on  Value=5.89e-01  SampleTime=-1
  Constant5 : Constant  Commented=on  Value=-1.47  SampleTime=-1
  Data Store Read : DataStoreRead  DataStoreName=MODEL  DataStoreElements=MODEL.OUTPUT.LATITUDE  IndexOptions=Index vector (dialog)  Indices=1  OutputSizes=1
  Data Store Read1 : DataStoreRead  DataStoreName=MODEL  DataStoreElements=MODEL.OUTPUT.LONGITUDE  IndexOptions=Index vector (dialog)  Indices=1  OutputSizes=1
  Data Store Read4 : DataStoreRead  Commented=on  DataStoreName=MODEL  DataStoreElements=MODEL.OUTPUT.PITCH  IndexOptions=Index vector (dialog)  Indices=1  OutputSizes=1
  Data Store Read5 : DataStoreRead  Commented=on  DataStoreName=CONTROL  DataStoreElements=CONTROL.OUTPUT.HEADING_NED  IndexOptions=Index vector (dialog)  Indices=1  OutputSizes=1
  Data Store Write : DataStoreWrite  Commented=on  DataStoreName=MODEL  DataStoreElements=MODEL.INPUT.LATITUDE  IndexOptions=Index vector (dialog)  Indices=1  OutputSizes=1
  Data Store Write1 : DataStoreWrite  Commented=on  DataStoreName=MODEL  DataStoreElements=MODEL.INPUT.LONGITUDE  IndexOptions=Index vector (dialog)  Indices=1  OutputSizes=1
  Data Store Write2 : DataStoreWrite  Commented=on  DataStoreName=MODEL  DataStoreElements=MODEL.INPUT.ALTITUDE  IndexOptions=Index vector (dialog)  Indices=1  OutputSizes=1
  Display1 : Display  Commented=on
  Display10 : Display
  Display11 : Display
  Display2 : Display  Commented=on
  Display3 : Display  Commented=on
  SimConnect Sink1 : SimConnectToolbox/SimConnect Sink  Commented=on  configurationIndex=0  connectionName=SimConnectSink  variables=|
      | PLANE ALTITUDE, FEET;
      | PLANE LATITUDE, RADIANS;
      | PLANE LONGITUDE, RADIANS;
      | PLANE PITCH DEGREES, RADIANS;
      | PLANE HEADING DEGREES TRUE, RADIANS;
      | ROTATION VELOCITY BODY X, FEET PER SECOND;
      | AILERON POSITION, POSITION;
      | AILERON TRIM PCT, PERCENT;
      settings: SourceProductName=SimConnect Toolbox
      mask Display:
      | % This is a new mask on top of the base mask.
      | % Use "View base mask" link below to see the base mask.
      | %port_label('input', 1, 'Rudder Trim', 'texmode', 'on')
      | port_label('input', 1, 'PLANE ALTITUDE, FEET', 'texmode', 'on')
      | port_label('input', 2, 'PLANE LATITUDE, RADIANS', 'texmode', 'on')
      | port_label('input', 3, 'PLANE LONGITUDE, RADIANS', 'texmode', 'on')
      | port_label('input', 4, 'PITCH DEGREES, RADIANS', 'texmode', 'on')
      | port_label('input', 5, 'HEADING DEGREES TRUE, RADIANS', 'texmode', 'on')
      | port_label('input', 6, 'VELOCITY BODY X, FEET PER SECOND', 'texmode', 'on')
      | port_label('input', 7, 'AILERON POSITION, POSITION', 'texmode', 'on')
      | port_label('input', 8, 'AILERON TRIM PCT, PERCENT OVER 100', 'texmode', 'on')
  SimConnect Source1 : SimConnectToolbox/SimConnect Source  Commented=on  configurationIndex=0  connectionName=SimConnectSource  variables=|
      | PLANE ALTITUDE, FEET;
      | PLANE LATITUDE, RADIANS;
      | PLANE LONGITUDE, RADIANS;
      settings: SourceProductName=SimConnect Toolbox
      mask Display:
      | % This is a new mask on top of the base mask.
      | % Use "View base mask" link below to see the base mask.
      | % port_label('output', 1, 'g', 'texmode', 'on')
      | port_label('output', 1, 'PLANE ALTITUDE, FEET', 'texmode', 'on')
      | port_label('output', 2, 'PLANE LATITUDE, RADIANS', 'texmode', 'on')
      | port_label('output', 3, 'PLANE LONGITUDE, RADIANS', 'texmode', 'on')
  wires:
  Data Store Read4/1 -> SimConnect Sink1/4
  Constant4/1 -> SimConnect Sink1/2
  Constant3/1 -> SimConnect Sink1/1
  Constant1/1 -> SimConnect Sink1/7
  Constant5/1 -> SimConnect Sink1/3
  Constant/1 -> SimConnect Sink1/6
  Data Store Read5/1 -> SimConnect Sink1/5
  Constant2/1 -> SimConnect Sink1/8
  SimConnect Source1/1 -> Display3/1, Data Store Write2/1
  SimConnect Source1/2 -> Display2/1, Data Store Write/1
  SimConnect Source1/3 -> Display1/1, Data Store Write1/1
  Data Store Read1/1 -> Display11/1
  Data Store Read/1 -> Display10/1

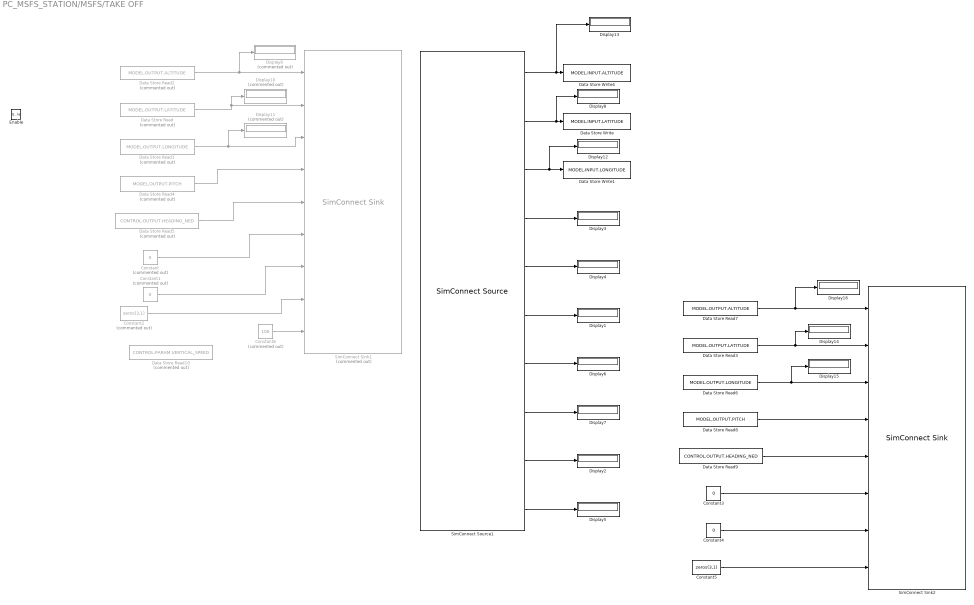
== system PC_MSFS_STATION/MSFS/TAKE OFF ==
  Enable : EnablePort
  Constant : Constant  Commented=on  Value=0  SampleTime=-1
  Constant1 : Constant  Commented=on  Value=0  SampleTime=-1
  Constant2 : Constant  Commented=on  Value=zeros(3,1)  SampleTime=-1
  Constant3 : Constant  Value=0  SampleTime=-1
  Constant4 : Constant  Value=0  SampleTime=-1
  Constant5 : Constant  Value=zeros(3,1)  SampleTime=-1
  Constant6 : Constant  Commented=on  Value=100  SampleTime=-1
  Data Store Read : DataStoreRead  Commented=on  DataStoreName=MODEL  DataStoreElements=MODEL.OUTPUT.LATITUDE  IndexOptions=Index vector (dialog)  Indices=1  OutputSizes=1
  Data Store Read1 : DataStoreRead  Commented=on  DataStoreName=MODEL  DataStoreElements=MODEL.OUTPUT.LONGITUDE  IndexOptions=Index vector (dialog)  Indices=1  OutputSizes=1
  Data Store Read10 : DataStoreRead  Commented=on  DataStoreName=CONTROL  DataStoreElements=CONTROL.PARAM.VERTICAL_SPEED  IndexOptions=Index vector (dialog)  Indices=1  OutputSizes=1
  Data Store Read2 : DataStoreRead  Commented=on  DataStoreName=MODEL  DataStoreElements=MODEL.OUTPUT.ALTITUDE  IndexOptions=Index vector (dialog)  Indices=1  OutputSizes=1
  Data Store Read3 : DataStoreRead  DataStoreName=MODEL  DataStoreElements=MODEL.OUTPUT.LATITUDE  IndexOptions=Index vector (dialog)  Indices=1  OutputSizes=1
  Data Store Read4 : DataStoreRead  Commented=on  DataStoreName=MODEL  DataStoreElements=MODEL.OUTPUT.PITCH  IndexOptions=Index vector (dialog)  Indices=1  OutputSizes=1
  Data Store Read5 : DataStoreRead  Commented=on  DataStoreName=CONTROL  DataStoreElements=CONTROL.OUTPUT.HEADING_NED  IndexOptions=Index vector (dialog)  Indices=1  OutputSizes=1
  Data Store Read6 : DataStoreRead  DataStoreName=MODEL  DataStoreElements=MODEL.OUTPUT.LONGITUDE  IndexOptions=Index vector (dialog)  Indices=1  OutputSizes=1
  Data Store Read7 : DataStoreRead  DataStoreName=MODEL  DataStoreElements=MODEL.OUTPUT.ALTITUDE  IndexOptions=Index vector (dialog)  Indices=1  OutputSizes=1
  Data Store Read8 : DataStoreRead  DataStoreName=MODEL  DataStoreElements=MODEL.OUTPUT.PITCH  IndexOptions=Index vector (dialog)  Indices=1  OutputSizes=1
  Data Store Read9 : DataStoreRead  DataStoreName=CONTROL  DataStoreElements=CONTROL.OUTPUT.HEADING_NED  IndexOptions=Index vector (dialog)  Indices=1  OutputSizes=1
  Data Store Write : DataStoreWrite  DataStoreName=MODEL  DataStoreElements=MODEL.INPUT.LATITUDE  IndexOptions=Index vector (dialog)  Indices=1  OutputSizes=1
  Data Store Write1 : DataStoreWrite  DataStoreName=MODEL  DataStoreElements=MODEL.INPUT.LONGITUDE  IndexOptions=Index vector (dialog)  Indices=1  OutputSizes=1
  Data Store Write4 : DataStoreWrite  DataStoreName=MODEL  DataStoreElements=MODEL.INPUT.ALTITUDE  IndexOptions=Index vector (dialog)  Indices=1  OutputSizes=1
  Display{1..8,12..16} (13 alike) : Display
  Display10 : Display  Commented=on
  Display11 : Display  Commented=on
  Display9 : Display  Commented=on
  SimConnect Sink1 : SimConnectToolbox/SimConnect Sink  Commented=on  configurationIndex=0  connectionName=SimConnectSink  variables=|
      | PLANE ALTITUDE, FEET;
      | PLANE LATITUDE, RADIANS;
      | PLANE LONGITUDE, RADIANS;
      | PLANE PITCH DEGREES, RADIANS;
      | PLANE HEADING DEGREES MAGNETIC, RADIANS;
      | ROTATION VELOCITY BODY X, FEET PER SECOND;
      | AILERON POSITION, POSITION;
      | AILERON TRIM PCT, PERCENT;
      | VERTICAL SPEED, FEET PER SECOND;
      settings: SourceProductName=SimConnect Toolbox
      mask Display:
      | % This is a new mask on top of the base mask.
      | % Use "View base mask" link below to see the base mask.
      | %port_label('input', 1, 'Rudder Trim', 'texmode', 'on')
      | port_label('input', 1, 'PLANE ALTITUDE, FEET', 'texmode', 'on')
      | port_label('input', 2, 'PLANE LATITUDE, RADIANS', 'texmode', 'on')
      | port_label('input', 3, 'PLANE LONGITUDE, RADIANS', 'texmode', 'on')
      | port_label('input', 4, 'PITCH DEGREES, RADIANS', 'texmode', 'on')
      | port_label('input', 5, 'HEADING DEGREES TRUE, RADIANS', 'texmode', 'on')
      | port_label('input', 6, 'VELOCITY BODY X, FEET PER SECOND', 'texmode', 'on')
      | port_label('input', 7, 'AILERON POSITION, POSITION', 'texmode', 'on')
      | port_label('input', 8, 'AILERON TRIM PCT, PERCENT OVER 100', 'texmode', 'on')
      | port_label('input', 9, 'VERTICAL SPEED, FEET PER SECOND', 'texmode', 'on')
  SimConnect Sink2 : SimConnectToolbox/SimConnect Sink  configurationIndex=0  connectionName=SimConnectSink  variables=|
      | PLANE ALTITUDE, FEET;
      | PLANE LATITUDE, RADIANS;
      | PLANE LONGITUDE, RADIANS;
      | PLANE PITCH DEGREES, RADIANS;
      | PLANE HEADING DEGREES MAGNETIC, RADIANS;
      | ROTATION VELOCITY BODY X, FEET PER SECOND;
      | AILERON POSITION, POSITION;
      | AILERON TRIM PCT, PERCENT;
      settings: SourceProductName=SimConnect Toolbox
      mask Display:
      | % This is a new mask on top of the base mask.
      | % Use "View base mask" link below to see the base mask.
      | %port_label('input', 1, 'Rudder Trim', 'texmode', 'on')
      | port_label('input', 1, 'PLANE ALTITUDE, FEET', 'texmode', 'on')
      | port_label('input', 2, 'PLANE LATITUDE, RADIANS', 'texmode', 'on')
      | port_label('input', 3, 'PLANE LONGITUDE, RADIANS', 'texmode', 'on')
      | port_label('input', 4, 'PITCH DEGREES, RADIANS', 'texmode', 'on')
      | port_label('input', 5, 'HEADING DEGREES TRUE, RADIANS', 'texmode', 'on')
      | port_label('input', 6, 'VELOCITY BODY X, FEET PER SECOND', 'texmode', 'on')
      | port_label('input', 7, 'AILERON POSITION, POSITION', 'texmode', 'on')
      | port_label('input', 8, 'AILERON TRIM PCT, PERCENT OVER 100', 'texmode', 'on')
  SimConnect Source1 : SimConnectToolbox/SimConnect Source  configurationIndex=0  connectionName=SimConnectSource  variables=|
      | PLANE ALTITUDE, FEET;
      | PLANE LATITUDE, RADIANS;
      | PLANE LONGITUDE, RADIANS;
      | ROTATION VELOCITY BODY X, FEET PER SECOND;
      | PLANE PITCH DEGREES, RADIANS;
      | PLANE HEADING DEGREES TRUE, RADIANS;
      | PLANE HEADING DEGREES MAGNETIC, RADIANS;
      | PLANE HEADING DEGREES GYRO, DEGREES;
      | AILERON POSITION, POSITION;
      | AILERON TRIM PCT, PERCENT OVER 100;
      settings: SourceProductName=SimConnect Toolbox
      mask Display:
      | % This is a new mask on top of the base mask.
      | % Use "View base mask" link below to see the base mask.
      | % port_label('output', 1, 'g', 'texmode', 'on')
      | port_label('output', 1, 'PLANE ALTITUDE, FEET', 'texmode', 'on')
      | port_label('output', 2, 'PLANE LATITUDE, RADIANS', 'texmode', 'on')
      | port_label('output', 3, 'PLANE LONGITUDE, RADIANS', 'texmode', 'on')
      | port_label('output', 4, 'VELOCITY BODY X, FEET PER SECOND', 'texmode', 'on')
      | port_label('output', 5, 'PITCH DEGREES, RADIANS', 'texmode', 'on')
      | port_label('output', 6, 'HEADING DEGREES TRUE, RADIANS', 'texmode', 'on')
      | port_label('output', 7, 'HEADING DEGREES MAGNETIC, RADIANS', 'texmode', 'on')
      | port_label('output', 8, 'HEADING DEGREES GYRO, DEGREES', 'texmode', 'on')
      | port_label('output', 9, 'AILERON POSITION, POSITION', 'texmode', 'on')
      | port_label('output', 10, 'AILERON TRIM PCT, PERCENT OVER 100', 'texmode', 'on')
  wires:
  Constant2/1 -> SimConnect Sink1/8
  SimConnect Source1/9 -> Display2/1
  Data Store Read5/1 -> SimConnect Sink1/5
  Constant/1 -> SimConnect Sink1/6
  Constant1/1 -> SimConnect Sink1/7
  SimConnect Source1/5 -> Display4/1
  SimConnect Source1/3 -> Display12/1, Data Store Write1/1
  SimConnect Source1/2 -> Display8/1, Data Store Write/1
  SimConnect Source1/8 -> Display7/1
  SimConnect Source1/6 -> Display1/1
  Data Store Read4/1 -> SimConnect Sink1/4
  SimConnect Source1/4 -> Display3/1
  SimConnect Source1/7 -> Display6/1
  SimConnect Source1/10 -> Display5/1
  Data Store Read2/1 -> SimConnect Sink1/1, Display9/1
  Data Store Read/1 -> Display10/1, SimConnect Sink1/2
  Data Store Read1/1 -> Display11/1, SimConnect Sink1/3
  SimConnect Source1/1 -> Display13/1, Data Store Write4/1
  Constant4/1 -> SimConnect Sink2/7
  Data Store Read9/1 -> SimConnect Sink2/5
  Data Store Read7/1 -> Display16/1, SimConnect Sink2/1
  Constant5/1 -> SimConnect Sink2/8
  Data Store Read8/1 -> SimConnect Sink2/4
  Data Store Read6/1 -> Display15/1, SimConnect Sink2/3
  Constant3/1 -> SimConnect Sink2/6
  Data Store Read3/1 -> Display14/1, SimConnect Sink2/2
  Constant6/1 -> SimConnect Sink1/9

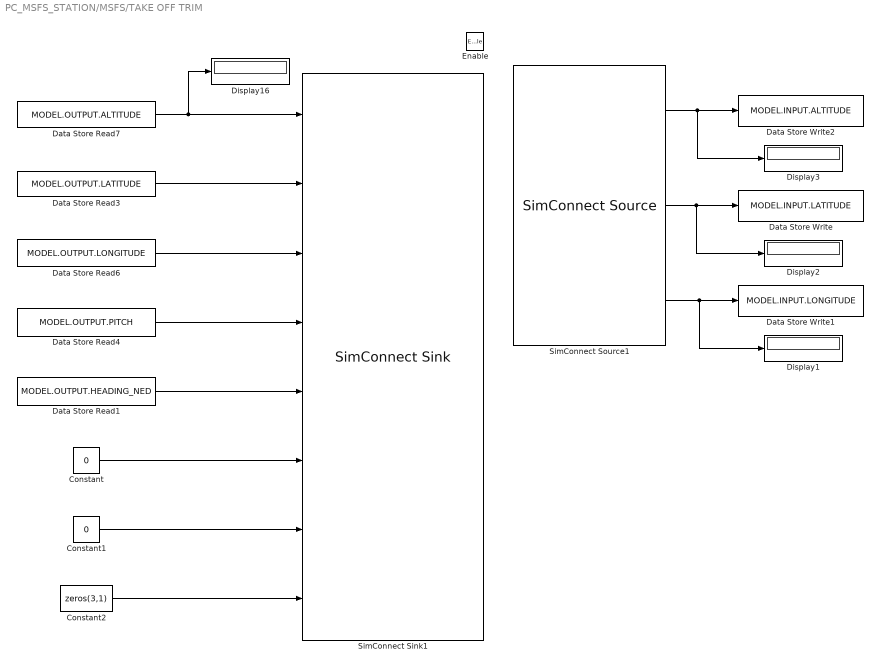
== system PC_MSFS_STATION/MSFS/TAKE OFF TRIM ==
  Enable : EnablePort
  Constant : Constant  Value=0  SampleTime=-1
  Constant1 : Constant  Value=0  SampleTime=-1
  Constant2 : Constant  Value=zeros(3,1)  SampleTime=-1
  Data Store Read1 : DataStoreRead  DataStoreName=MODEL  DataStoreElements=MODEL.OUTPUT.HEADING_NED  IndexOptions=Index vector (dialog)  Indices=1  OutputSizes=1
  Data Store Read3 : DataStoreRead  DataStoreName=MODEL  DataStoreElements=MODEL.OUTPUT.LATITUDE  IndexOptions=Index vector (dialog)  Indices=1  OutputSizes=1
  Data Store Read4 : DataStoreRead  DataStoreName=MODEL  DataStoreElements=MODEL.OUTPUT.PITCH  IndexOptions=Index vector (dialog)  Indices=1  OutputSizes=1
  Data Store Read6 : DataStoreRead  DataStoreName=MODEL  DataStoreElements=MODEL.OUTPUT.LONGITUDE  IndexOptions=Index vector (dialog)  Indices=1  OutputSizes=1
  Data Store Read7 : DataStoreRead  DataStoreName=MODEL  DataStoreElements=MODEL.OUTPUT.ALTITUDE  IndexOptions=Index vector (dialog)  Indices=1  OutputSizes=1
  Data Store Write : DataStoreWrite  DataStoreName=MODEL  DataStoreElements=MODEL.INPUT.LATITUDE  IndexOptions=Index vector (dialog)  Indices=1  OutputSizes=1
  Data Store Write1 : DataStoreWrite  DataStoreName=MODEL  DataStoreElements=MODEL.INPUT.LONGITUDE  IndexOptions=Index vector (dialog)  Indices=1  OutputSizes=1
  Data Store Write2 : DataStoreWrite  DataStoreName=MODEL  DataStoreElements=MODEL.INPUT.ALTITUDE  IndexOptions=Index vector (dialog)  Indices=1  OutputSizes=1
  Display{1..3,16} (4 alike) : Display
  SimConnect Sink1 : SimConnectToolbox/SimConnect Sink  configurationIndex=0  connectionName=SimConnectSink  variables=|
      | PLANE ALTITUDE, FEET;
      | PLANE LATITUDE, RADIANS;
      | PLANE LONGITUDE, RADIANS;
      | PLANE PITCH DEGREES, RADIANS;
      | PLANE HEADING DEGREES TRUE, RADIANS;
      | ROTATION VELOCITY BODY X, FEET PER SECOND;
      | AILERON POSITION, POSITION;
      | AILERON TRIM PCT, PERCENT;
      settings: SourceProductName=SimConnect Toolbox
      mask Display:
      | % This is a new mask on top of the base mask.
      | % Use "View base mask" link below to see the base mask.
      | %port_label('input', 1, 'Rudder Trim', 'texmode', 'on')
      | port_label('input', 1, 'PLANE ALTITUDE, FEET', 'texmode', 'on')
      | port_label('input', 2, 'PLANE LATITUDE, RADIANS', 'texmode', 'on')
      | port_label('input', 3, 'PLANE LONGITUDE, RADIANS', 'texmode', 'on')
      | port_label('input', 4, 'PITCH DEGREES, RADIANS', 'texmode', 'on')
      | port_label('input', 5, 'HEADING DEGREES TRUE, RADIANS', 'texmode', 'on')
      | port_label('input', 6, 'VELOCITY BODY X, FEET PER SECOND', 'texmode', 'on')
      | port_label('input', 7, 'AILERON POSITION, POSITION', 'texmode', 'on')
      | port_label('input', 8, 'AILERON TRIM PCT, PERCENT OVER 100', 'texmode', 'on')
  SimConnect Source1 : SimConnectToolbox/SimConnect Source  configurationIndex=0  connectionName=SimConnectSource  variables=|
      | PLANE ALTITUDE, FEET;
      | PLANE LATITUDE, RADIANS;
      | PLANE LONGITUDE, RADIANS;
      settings: SourceProductName=SimConnect Toolbox
      mask Display:
      | % This is a new mask on top of the base mask.
      | % Use "View base mask" link below to see the base mask.
      | % port_label('output', 1, 'g', 'texmode', 'on')
      | port_label('output', 1, 'PLANE ALTITUDE, FEET', 'texmode', 'on')
      | port_label('output', 2, 'PLANE LATITUDE, RADIANS', 'texmode', 'on')
      | port_label('output', 3, 'PLANE LONGITUDE, RADIANS', 'texmode', 'on')
  wires:
  Data Store Read7/1 -> SimConnect Sink1/1, Display16/1
  SimConnect Source1/2 -> Data Store Write/1, Display2/1
  SimConnect Source1/1 -> Display3/1, Data Store Write2/1
  SimConnect Source1/3 -> Display1/1, Data Store Write1/1
  Data Store Read3/1 -> SimConnect Sink1/2
  Data Store Read6/1 -> SimConnect Sink1/3
  Data Store Read1/1 -> SimConnect Sink1/5
  Constant1/1 -> SimConnect Sink1/7
  Constant/1 -> SimConnect Sink1/6
  Constant2/1 -> SimConnect Sink1/8
  Data Store Read4/1 -> SimConnect Sink1/4
